simulink model "ready_to_build_controller"  (R2024a)
settings: Solver=FixedStepAuto  StartTime=0.0  StopTime=inf  RelTol=1e-3
libraries: robotlib x3, cstblocks x1
settings Model: Creator=stanleychiu  LastModifiedBy=stanleychiu
settings OptimizationCC: EnhancedBackFolding=on  PassReuseOutputArgsAs=Individual arguments  ZeroExternalMemoryAtStartup=off  ZeroInternalMemoryAtStartup=off  MaxStackSize=64  OptimizeBlockOrder=speed  DifferentSizesBufferReuse=on  OptimizationCustomize=off  EfficientTunableParamExpr=on
settings DebuggingCC: ParameterTunabilityLossMsg=error
settings HardwareCC: ProdBitPerPointer=32  ProdBitPerSizeT=32  ProdBitPerPtrDiffT=32  ProdLargestAtomicFloat=None  ProdIntDivRoundTo=Undefined  ProdEndianess=Unspecified  ProdWordSize=32  ProdHWDeviceType=Generic->Unspecified (assume 32-bit Generic)  UseEmbeddedCoderFeatures=off
settings SFSimCC: MATLABDynamicMemAlloc=off
settings RTWCC: Description=Embedded Coder  SystemTargetFile=ert.tlc  HardwareBoard=Robot Operating System (ROS)  TLCOptions="-aInlineSetEventsForThisBaseRateFcn=TLC_FALSE -aSuppressMultiTaskScheduler=TLC_FALSE  -aRateBasedStepFcn=0"  TemplateMakefile=ert_default_tmf  Toolchain=Catkin  TargetLang=C++
settings CodeAppCC: ForceParamTrailComments=on  IgnoreCustomStorageClasses=off  OperatorAnnotations=on  SimulinkDataObjDesc=on  SFDataObjDesc=on  InsertBlockDesc=on
settings ERTTargetCC: SupportNonInlinedSFcns=on

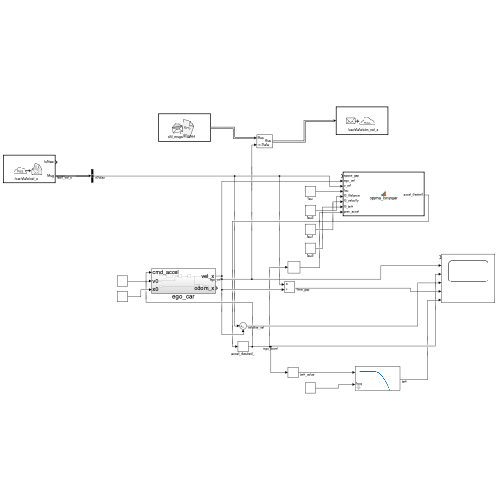
[thumbnail: Simulink's stored preview of the top-level diagram]
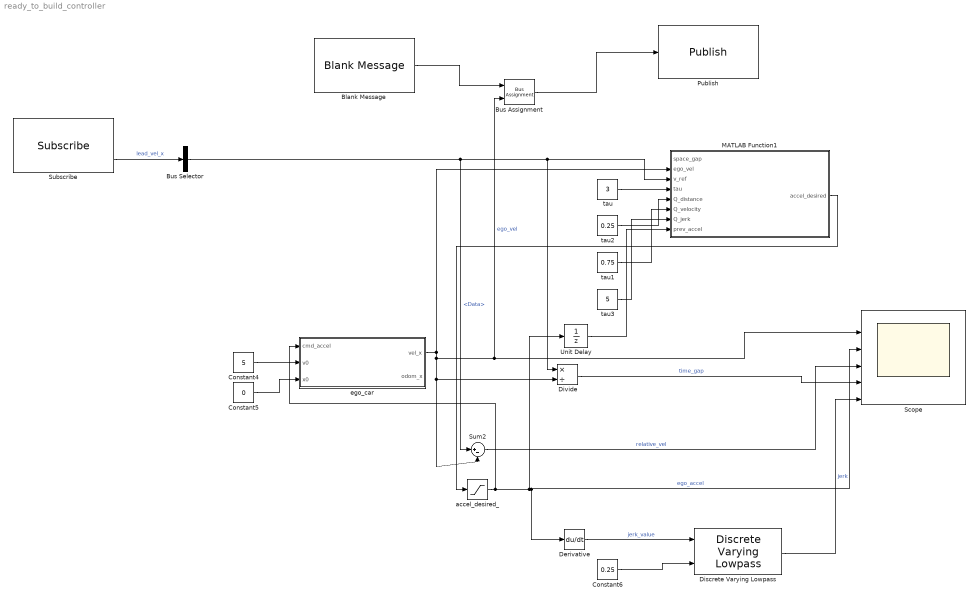
== system ready_to_build_controller ==
  Blank Message : robotlib/Blank Message  messageClass=Message  entityType=std_msgs/Float64  messageType=std_msgs/Float64  SampleTime=inf  legacyBusStruct=off
  Bus Assignment : BusAssignment  AssignedSignals=Data
  Bus Selector : BusSelector  OutputSignals=Data
  Constant4 : Constant  Value=5
  Constant5 : Constant  Value=0
  Constant6 : Constant  Value=0.25
  Derivative : Derivative
  Discrete Varying Lowpass : cstblocks/Linear Parameter Varying/Discrete Varying Lowpass  N=1  w0=0  Ts=0.1
  Divide : Product  Inputs=*/
  MATLAB Function1 : MATLAB Function  TreatAsAtomicUnit=on
  Publish : robotlib/Publish  topicSource=Specify your own  topic=/car/state/sim_vel_x  messageType=std_msgs/Float64  legacyBusStruct=off  messageQueueLength=1
  Scope : Scope  NumInputPorts=6
  Subscribe : robotlib/Subscribe  topicSource=Specify your own  topic=/car/state/vel_x  messageType=std_msgs/Float64  SampleTime=-1  legacyBusStruct=off  messageQueueLength=1
  Sum2 : Sum  Inputs=|+-
  Unit Delay : UnitDelay  SampleTime=-1  HasFrameUpgradeWarning=on
  accel_desired_ : Saturate  UpperLimit=20  LowerLimit=-20
  ego_car : Subsystem
  tau : Constant  Value=3
  tau1 : Constant  Value=0.75
  tau2 : Constant  Value=0.25
  tau3 : Constant  Value=5
  wires:
  Discrete Varying Lowpass/1 -> Scope/6  "jerk"
  MATLAB Function1/1(accel_desired) -> accel_desired_/1
  Constant6/1 -> Discrete Varying Lowpass/2
  Derivative/1 -> Discrete Varying Lowpass/1  "jerk_value"
  Divide/1 -> Scope/5  "time_gap"
  Unit Delay/1 -> MATLAB Function1/8(prev_accel)
  tau2/1 -> MATLAB Function1/5(Q_distance)
  Sum2/1 -> Scope/4  "relative_vel"
  tau1/1 -> MATLAB Function1/6(Q_velocity)
  accel_desired_/1 -> Derivative/1, Scope/3, Unit Delay/1, ego_car/1(cmd_accel)  "ego_accel"
  Constant5/1 -> ego_car/3(x0)
  Constant4/1 -> ego_car/2(v0)
  tau/1 -> MATLAB Function1/4(tau)
  ego_car/1(vel_x) -> Sum2/2, Divide/2, Bus Assignment/2, Scope/2, MATLAB Function1/2(ego_vel)  "ego_vel"
  tau3/1 -> MATLAB Function1/7(Q_jerk)
  Bus Assignment/1 -> Publish/1
  Blank Message/1 -> Bus Assignment/1
  Subscribe/2 -> Bus Selector/1  "lead_vel_x"
  Bus Selector/1 -> Sum2/1, Divide/1, MATLAB Function1/3(v_ref)  "<Data>"

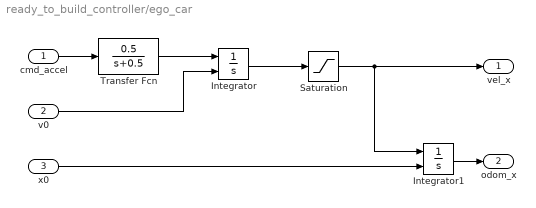
== system ready_to_build_controller/ego_car ==
  cmd_accel : Inport
  v0 : Inport  Port=2
  x0 : Inport  Port=3
  Integrator : Integrator  InitialConditionSource=external
  Integrator1 : Integrator  InitialConditionSource=external
  Saturation : Saturate  UpperLimit=80  LowerLimit=0
  Transfer Fcn : TransferFcn  Numerator=[0.5]  Denominator=[1 0.5]
  vel_x : Outport
  odom_x : Outport  Port=2
  wires:
  v0/1 -> Integrator/2
  cmd_accel/1 -> Transfer Fcn/1
  Transfer Fcn/1 -> Integrator/1
  Integrator1/1 -> odom_x/1
  Integrator/1 -> Saturation/1
  x0/1 -> Integrator1/2
  Saturation/1 -> vel_x/1, Integrator1/1

== matlab function ready_to_build_controller/MATLAB Function1 ==
  data: space_gap input; accel_desired output; ego_vel input; v_ref input; tau input; Q_distance input; Q_velocity input; Q_jerk input; prev_accel input
function accel_desired = optimal_controller(space_gap, ego_vel, v_ref, tau, Q_distance, Q_velocity, Q_jerk, prev_accel)
    % Inputs:
    % space_gap: Current gap between the ego vehicle and the lead vehicle
    % ego_vel: Current velocity of the ego vehicle
    % v_ref: Reference velocity (desired velocity or lead vehicle velocity)
    % tau: Time gap (constant time gap parameter)
    % Q_distance: Weight for space gap penalty
    % Q_velocity: Weight for velocity penalty
    % Q_jerk: Weight for jerk penalty
    % prev_accel: Previous acceleration (used to compute jerk)

    % Define the desired space gap based on the time gap
    desired_gap = ego_vel * tau;

    % Set bounds for acceleration (e.g., physical limits of the vehicle)
    accel_min = -3;   % Minimum allowed acceleration (e.g., maximum braking)
    accel_max = 1.5;  % Maximum allowed acceleration (e.g., maximum acceleration)

    % Compute the optimal acceleration analytically
    numerator = Q_velocity * (v_ref - ego_vel) + Q_jerk * prev_accel;
    denominator = Q_velocity + Q_jerk;

    accel_opt = numerator / denominator;

    % Clip the acceleration to lie within the allowed bounds
    accel_desired = max(accel_min, min(accel_opt, accel_max));
end
